simulink model "TwoScaleSimulation"  (R2021b)
settings: Solver=ode15s  StartTime=0.0  StopTime=1440  RelTol=1e-5
model workspace (MAT data in the model file):
  K_ACTH_StARp37 = 21.62
  k21 = 3080
  k_ACORT = 44.5
  k_StARp37 = 0.778
  ke = 0.099
  mu_StARp37 = 19.8
settings Model: Creator=Mahdi  LastModifiedBy=Mahdi
settings SolverCC: AlgebraicLoopSolver=TrustRegion
settings DebuggingCC: SFMachineParentedDataDiag=warning

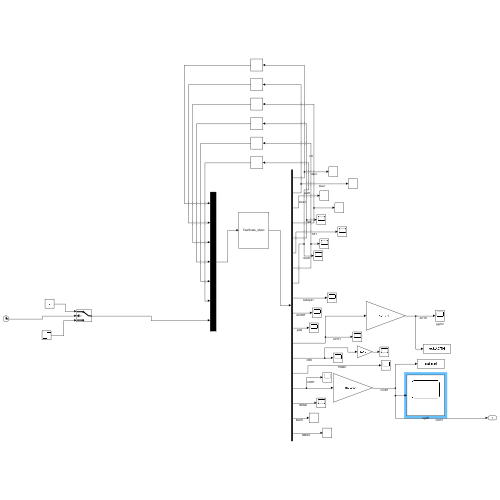
[thumbnail: Simulink's stored preview of the top-level diagram]
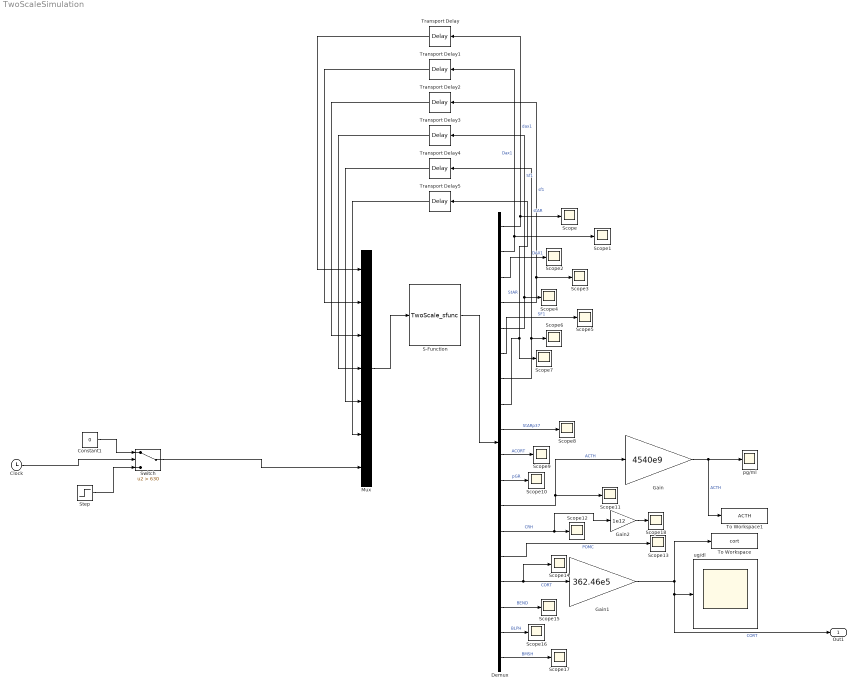
== system TwoScaleSimulation ==
  Clock : Clock
  Constant1 : Constant  Value=0
  Demux : Demux  Outputs=18
  Gain : Gain  Gain=4540e9
  Gain1 : Gain  Gain=362.46e5
  Gain2 : Gain  Gain=1e12
  Mux : Mux  Inputs=7
  S-Function : S-Function  FunctionName=TwoScale_sfunc  SFunctionDeploymentMode=off  EnableBusSupport=off
  Scope{,1..18} (19 alike) : Scope
  Step : Step  Time=600  SampleTime=0
  Switch : Switch  Criteria=u2 > Threshold  Threshold=630
  To Workspace : ToWorkspace  VariableName=cort  SampleTime=0.1
  To Workspace1 : ToWorkspace  VariableName=ACTH  SampleTime=0.1
  Transport Delay : TransportDelay  DelayTime=2.79
  Transport Delay1 : TransportDelay  DelayTime=1.4
  Transport Delay2 : TransportDelay  DelayTime=14.75
  Transport Delay3 : TransportDelay  DelayTime=1.38
  Transport Delay4 : TransportDelay  DelayTime=5.58
  Transport Delay5 : TransportDelay
  pg/ml : Scope
  ug/dl : Scope
  Out1 : Outport
  wires:
  Demux/10 -> Scope9/1  "ACORT"
  Demux/6 -> Scope5/1  "SF1"
  Demux/7 -> Transport Delay4/1, Scope6/1  "stAR"
  Demux/2 -> Transport Delay1/1, Scope1/1  "Dax1"
  Demux/4 -> Transport Delay2/1, Scope3/1  "sf1"
  Mux/1 -> S-Function/1
  Transport Delay4/1 -> Mux/5
  Transport Delay1/1 -> Mux/2
  Transport Delay/1 -> Mux/1
  Demux/11 -> Scope10/1  "pGR"
  Transport Delay5/1 -> Mux/6
  Demux/8 -> Scope7/1, Transport Delay5/1  "StAR"
  Demux/9 -> Scope8/1  "StARp37"
  S-Function/1 -> Demux/1
  Transport Delay3/1 -> Mux/4
  Demux/3 -> Scope2/1  "DAX1"
  Demux/1 -> Transport Delay/1, Scope/1  "dax1"
  Demux/5 -> Transport Delay3/1, Scope4/1  "Sf1"
  Transport Delay2/1 -> Mux/3
  Demux/12 -> Scope11/1, Gain/1  "ACTH"
  Demux/13 -> Gain2/1, Scope12/1  "CRH"
  Demux/14 -> Scope13/1  "POMC"
  Demux/15 -> Scope14/1, Gain1/1  "CORT"
  Gain/1 -> To Workspace1/1, pg/ml/1  "ACTH"
  Gain1/1 -> ug/dl/1, Out1/1, To Workspace/1  "CORT"
  Switch/1 -> Mux/7
  Demux/16 -> Scope15/1  "BEND"
  Demux/17 -> Scope16/1  "BLPH"
  Demux/18 -> Scope17/1  "BMSH"
  Gain2/1 -> Scope18/1
  Step/1 -> Switch/3
  Constant1/1 -> Switch/1
  Clock/1 -> Switch/2
